simulink model "reactor_withMLcontroller"  (R2018a)
settings: Solver=VariableStepAuto  StartTime=0.0  StopTime=100.0  RelTol=1e-3
settings Model: Creator=Arefin Mahin  LastModifiedBy=Arefin Mahin

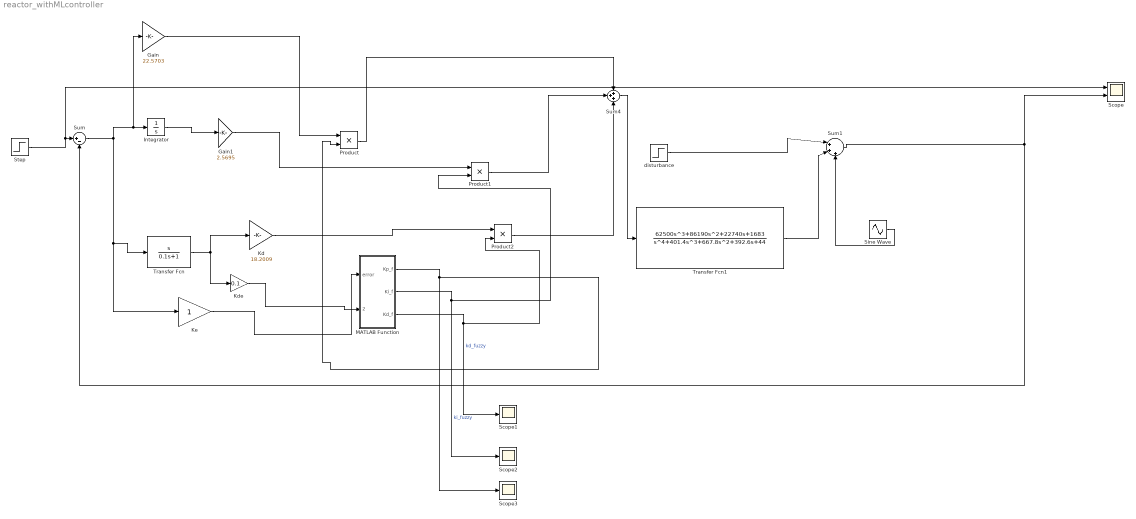
== system reactor_withMLcontroller ==
  Gain : Gain  Gain=22.5703
  Gain1 : Gain  Gain=2.5695
  Integrator : Integrator
  Kd : Gain  Gain=18.2009
  Kde : Gain  Gain=0.1
  Ke : Gain
  MATLAB Function : MATLAB Function  TreatAsAtomicUnit=on
  Product : Product
  Product1 : Product
  Product2 : Product
  Scope : Scope  NumInputPorts=2
  Scope1 : Scope
  Scope2 : Scope
  Scope3 : Scope
  Sine Wave : Sin  Amplitude=0.4  SampleTime=0
  Step : Step  SampleTime=0
  Sum : Sum  Inputs=|+-
  Sum1 : Sum  Inputs=|+++
  Sum4 : Sum  Inputs=3
  Transfer Fcn : TransferFcn  Numerator=[1 0]  Denominator=[0.1 1]
  Transfer Fcn1 : TransferFcn  Numerator=[62500 86190 22740 1683]  Denominator=[1 401.4 667.8 392.6 44]
  disturbance : Step  Time=15  SampleTime=0
  wires:
  Ke/1 -> MATLAB Function/1(error)
  Sum4/1 -> Transfer Fcn1/1
  Kd/1 -> Product2/1
  Product2/1 -> Sum4/3
  MATLAB Function/3(Kd_f) -> Scope1/1, Product2/2  "kd_fuzzy"
  Product/1 -> Sum4/1
  disturbance/1 -> Sum1/1
  Product1/1 -> Sum4/2
  MATLAB Function/1(Kp_f) -> Scope3/1, Product/2
  Gain1/1 -> Product1/1
  Kde/1 -> MATLAB Function/2(d_error)
  Gain/1 -> Product/1
  Transfer Fcn1/1 -> Sum1/2
  Sum1/1 -> Scope/2, Sum/2
  Transfer Fcn/1 -> Kde/1, Kd/1
  Step/1 -> Scope/1, Sum/1
  Integrator/1 -> Gain1/1
  MATLAB Function/2(Ki_f) -> Scope2/1, Product1/2  "ki_fuzzy"
  Sum/1 -> Ke/1, Transfer Fcn/1, Gain/1, Integrator/1
  Sine Wave/1 -> Sum1/3

== matlab function reactor_withMLcontroller/MATLAB Function ==
  settings: updateMethod=DISCRETE
  data: error input; Kp_f output; d_error input; Ki_f output; Kd_f output
function [Kp_f, Ki_f, Kd_f] = fcn(error, d_error)
       %#codegen
       persistent W1 b1 W2 b2 W3 b3 loaded
       if isempty(loaded)
           d  = coder.load('nn_weights.mat');
           W1 = d.fc1_weight;  b1 = d.fc1_bias(:);
           W2 = d.fc2_weight;  b2 = d.fc2_bias(:);
           W3 = d.fc3_weight;  b3 = d.fc3_bias(:);
           loaded = true;
       end
       x = [error; d_error];
       h1 = tanh(W1 * x  + b1);
       h2 = tanh(W2 * h1 + b2);
       y  = 1 ./ (1 + exp(-(W3 * h2 + b3)));
       Kp_f = y(1);
       Ki_f = y(2);
       Kd_f = y(3);
   end
